simulink model "Q10"  (R2024a)
settings: Solver=FixedStepAuto  StartTime=0.0  StopTime=0.1  FixedStep=1e-5  RelTol=1e-3
undefined symbols (not defined in the file): C, G, H, k, P, Ts
settings Model: Creator=psatt  LastModifiedBy=ali
settings RTWCC: GPUComputeCapability=3.5

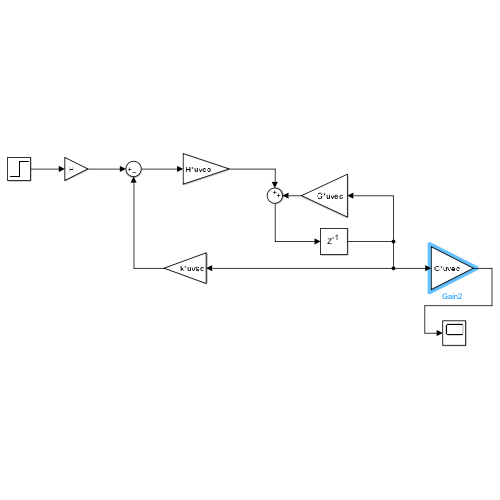
[thumbnail: Simulink's stored preview of the top-level diagram]
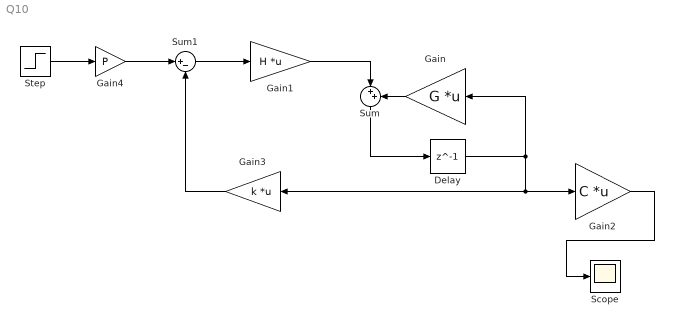
== system Q10 ==
  Delay : Delay  DelayLength=1  SampleTime=Ts
  Gain : Gain  Gain=G  Multiplication=Matrix(K*u) (u vector)
  Gain1 : Gain  Gain=H  Multiplication=Matrix(K*u) (u vector)
  Gain2 : Gain  Gain=C  Multiplication=Matrix(K*u) (u vector)
  Gain3 : Gain  Gain=k  Multiplication=Matrix(K*u) (u vector)
  Gain4 : Gain  Gain=P
  Scope : Scope
  Step : Step  Time=0  After=0.002  SampleTime=0
  Sum : Sum  Inputs=|++
  Sum1 : Sum  Inputs=|+-
  wires:
  Gain/1 -> Sum/2
  Sum/1 -> Delay/1
  Gain1/1 -> Sum/1
  Delay/1 -> Gain2/1, Gain3/1, Gain/1
  Gain3/1 -> Sum1/2
  Sum1/1 -> Gain1/1
  Gain2/1 -> Scope/1
  Step/1 -> Gain4/1
  Gain4/1 -> Sum1/1
